simulink model "BMS_v1"  (R2024b)
settings: Solver=VariableStepAuto  StartTime=0.0  StopTime=1000  RelTol=1e-3  AbsTol=1e-3  EnableMultiTasking=on
libraries: fl_lib x30, nesl_utility x20, batt_lib x4
(part 2 of 2)

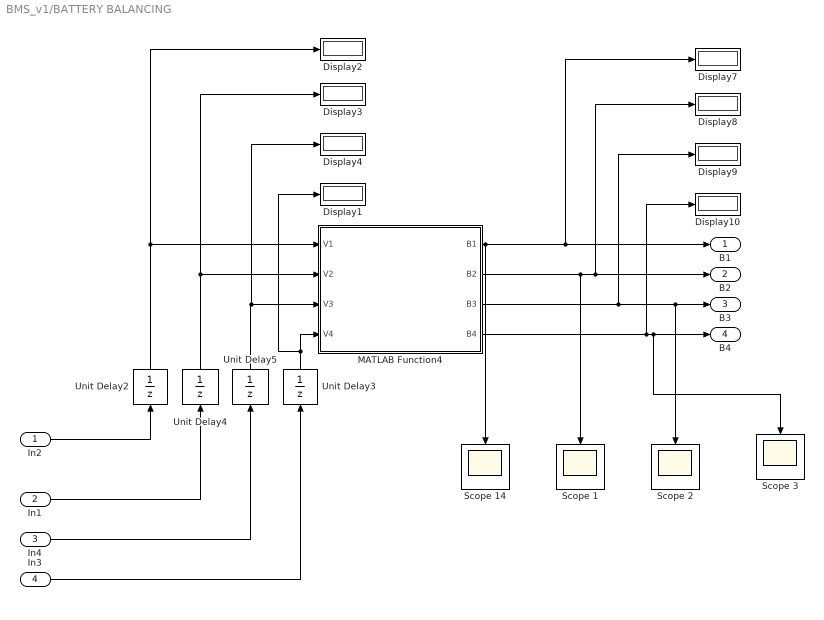
== system BMS_v1/BATTERY BALANCING ==
  In2 : Inport
  In1 : Inport  Port=2
  In4 : Inport  Port=3
  In3 : Inport  Port=4
  Display{1..4,7..10} (8 alike) : Display
  MATLAB Function4 : MATLAB Function  TreatAsAtomicUnit=on  SystemSampleTime=1
  Scope {1..3,14} (4 alike) : Scope
  Unit Delay{2..5} (4 alike) : UnitDelay  InitialCondition=4  HasFrameUpgradeWarning=on
  B1 : Outport
  B2 : Outport  Port=2
  B3 : Outport  Port=3
  B4 : Outport  Port=4
  wires:
  Unit Delay2/1 -> Display2/1, MATLAB Function4/1(V1)
  Unit Delay5/1 -> Display4/1, MATLAB Function4/3(V3)
  MATLAB Function4/4(B4) -> Scope 3/1, B4/1, Display10/1
  Unit Delay4/1 -> Display3/1, MATLAB Function4/2(V2)
  MATLAB Function4/2(B2) -> B2/1, Display8/1, Scope 1/1
  MATLAB Function4/1(B1) -> B1/1, Display7/1, Scope 14/1
  MATLAB Function4/3(B3) -> Scope 2/1, B3/1, Display9/1
  Unit Delay3/1 -> MATLAB Function4/4(V4), Display1/1
  In4/1 -> Unit Delay5/1
  In2/1 -> Unit Delay2/1
  In3/1 -> Unit Delay3/1
  In1/1 -> Unit Delay4/1

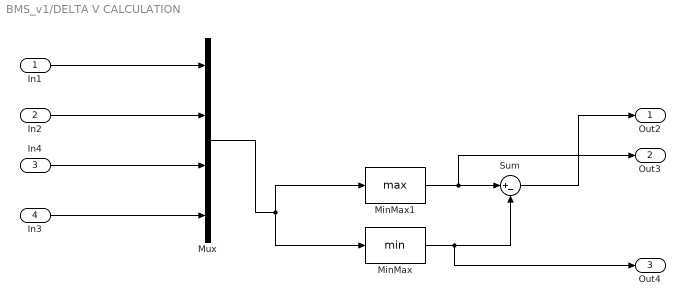
== system BMS_v1/DELTA V CALCULATION ==
  In1 : Inport
  In2 : Inport  Port=2
  In4 : Inport  Port=3
  In3 : Inport  Port=4
  MinMax : MinMax
  MinMax1 : MinMax  Function=max
  Mux : Mux
  Sum : Sum  Inputs=|+-
  Out2 : Outport
  Out3 : Outport  Port=2
  Out4 : Outport  Port=3
  wires:
  In3/1 -> Mux/4
  Mux/1 -> MinMax/1, MinMax1/1
  In1/1 -> Mux/1
  MinMax1/1 -> Out3/1, Sum/1
  MinMax/1 -> Out4/1, Sum/2
  In2/1 -> Mux/2
  Sum/1 -> Out2/1
  In4/1 -> Mux/3

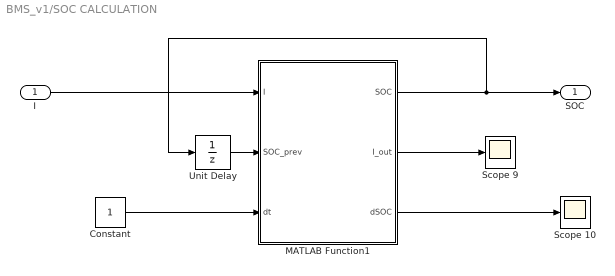
== system BMS_v1/SOC CALCULATION ==
  I : Inport
  Constant : Constant
  MATLAB Function1 : MATLAB Function  TreatAsAtomicUnit=on
  Scope 10 : Scope
  Scope 9 : Scope
  Unit Delay : UnitDelay  InitialCondition=0.9  HasFrameUpgradeWarning=on
  SOC : Outport
  wires:
  MATLAB Function1/1(SOC) -> SOC/1, Unit Delay/1
  MATLAB Function1/2(I_out) -> Scope 9/1
  MATLAB Function1/3(dSOC) -> Scope 10/1
  Constant/1 -> MATLAB Function1/3(dt)
  Unit Delay/1 -> MATLAB Function1/2(SOC_prev)
  I/1 -> MATLAB Function1/1(I)

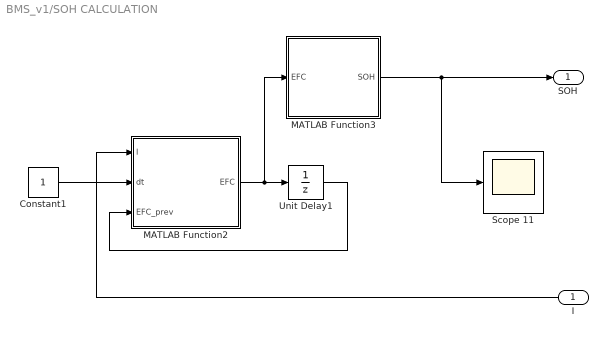
== system BMS_v1/SOH CALCULATION ==
  I : Inport
  Constant1 : Constant
  MATLAB Function2 : MATLAB Function  TreatAsAtomicUnit=on
  MATLAB Function3 : MATLAB Function  TreatAsAtomicUnit=on
  Scope 11 : Scope
  Unit Delay1 : UnitDelay  InitialCondition=0.9  HasFrameUpgradeWarning=on
  SOH : Outport
  wires:
  MATLAB Function2/1(EFC) -> MATLAB Function3/1(EFC), Unit Delay1/1
  MATLAB Function3/1(SOH) -> SOH/1, Scope 11/1
  Constant1/1 -> MATLAB Function2/2(dt)
  Unit Delay1/1 -> MATLAB Function2/3(EFC_prev)
  I/1 -> MATLAB Function2/1(I)

== matlab function BMS_v1/MATLAB Function3 ==
  data: Fault input; FaultCode input; State output; Reset input; System_Enable input; Charge_Request input; Discharge_Request input; Main_Contactor output; Precharge_Contactor output; Charge_Enable output; Discharge_Enable output; Fault_Action output; Precharge_Complete input; Time input
function [State, Main_Contactor, Precharge_Contactor, ...
          Charge_Enable, Discharge_Enable, Fault_Action] = ...
    BMS_State_Machine(Fault, FaultCode, Reset, System_Enable, ...
                      Charge_Request, Discharge_Request, ...
                      Precharge_Complete, Time)

% ============================================================
% BMS STATE MACHINE
%
% 0 = OFF
% 1 = INITIALIZE
% 2 = PRECHARGE
% 3 = IDLE
% 4 = CHARGING
% 5 = DISCHARGING
% 6 = FAULT
%
% Fault_Action:
% 0 = NORMAL
% 1 = WARNING / IMBALANCE
% 2 = CHARGE DISABLED
% 3 = DISCHARGE DISABLED
% 4 = CRITICAL FAULT
%
% FaultCode bits:
%
% 1   = Over-Voltage
% 2   = Under-Voltage
% 4   = Over-Current
% 8   = Over-Temperature
% 16  = Under-Temperature
% 32  = Cell Imbalance
% 64  = Low SOC
% 128 = Severe Fault
% 256 = Main Contactor Fault
% 512 = Precharge Contactor Fault
% ============================================================

persistent state
persistent precharge_start_time
persistent precharge_timeout_fault

if isempty(state)
    state = 0;
end

if isempty(precharge_start_time)
    precharge_start_time = 0;
end

if isempty(precharge_timeout_fault)
    precharge_timeout_fault = 0;
end

% ------------------------------------------------------------
% DEFAULT OUTPUTS
% ------------------------------------------------------------

State = 0;
Main_Contactor = 0;
Precharge_Contactor = 0;
Charge_Enable = 0;
Discharge_Enable = 0;
Fault_Action = 0;

% ------------------------------------------------------------
% FAULT CODE DECODING
% ------------------------------------------------------------

% Fault Manager uses uint16 because FaultCode can exceed 255
FC = uint16(FaultCode);

% Protection faults
OV   = bitand(FC,uint16(1))   ~= 0;
UV   = bitand(FC,uint16(2))   ~= 0;
OC   = bitand(FC,uint16(4))   ~= 0;
OT   = bitand(FC,uint16(8))   ~= 0;
UT   = bitand(FC,uint16(16))  ~= 0;
IMB  = bitand(FC,uint16(32))  ~= 0;
LSOC = bitand(FC,uint16(64))  ~= 0;
SEV  = bitand(FC,uint16(128)) ~= 0;

% Contactor diagnostic faults
MAIN_CONT_F  = bitand(FC,uint16(256)) ~= 0;
PRECH_CONT_F = bitand(FC,uint16(512)) ~= 0;

% ------------------------------------------------------------
% FAULT CLASSIFICATION
% ------------------------------------------------------------

if precharge_timeout_fault == 1

    % Latched precharge timeout
    Fault_Action = 4;

elseif Fault == 0

    Fault_Action = 0;

elseif SEV || OC || MAIN_CONT_F || PRECH_CONT_F

    % Critical faults
    Fault_Action = 4;

elseif OV || OT || UT

    % Charging prohibited
    Fault_Action = 2;

elseif UV || LSOC

    % Discharging prohibited
    Fault_Action = 3;

elseif IMB

    % Warning / balancing condition
    Fault_Action = 1;

else

    % Unknown fault = fail safe
    Fault_Action = 4;

end

% ============================================================
% STATE MACHINE
% ============================================================

switch state

    % ========================================================
    % STATE 0 : OFF
    % ========================================================

    case 0

        Main_Contactor = 0;
        Precharge_Contactor = 0;
        Charge_Enable = 0;
        Discharge_Enable = 0;

        precharge_start_time = 0;

        % Clear old timeout fault when system is completely OFF
        precharge_timeout_fault = 0;

        if System_Enable == 1

            state = 1;

        end


    % ========================================================
    % STATE 1 : INITIALIZE
    % ========================================================

    case 1

        Main_Contactor = 0;
        Precharge_Contactor = 0;
        Charge_Enable = 0;
        Discharge_Enable = 0;

        if Fault ~= 0

            state = 6;

        elseif precharge_timeout_fault == 1

            state = 6;

        else

            % Start precharge
            state = 2;

            % Record exact simulation time
            precharge_start_time = Time;

        end


    % ========================================================
    % STATE 2 : PRECHARGE
    % ========================================================

    case 2

        Precharge_Contactor = 1;
        Main_Contactor = 0;

        Charge_Enable = 0;
        Discharge_Enable = 0;

        % ----------------------------------------------------
        % CRITICAL FAULT DURING PRECHARGE
        % ----------------------------------------------------

        if Fault_Action == 4

            Precharge_Contactor = 0;
            Main_Contactor = 0;

            state = 6;

        % ----------------------------------------------------
        % PRECHARGE TIMEOUT
        % ----------------------------------------------------

        elseif (Time - precharge_start_time) >= 3

            Precharge_Contactor = 0;
            Main_Contactor = 0;

            % Latch timeout fault
            precharge_timeout_fault = 1;

            Fault_Action = 4;

            state = 6;

        % ----------------------------------------------------
        % PRECHARGE SUCCESS
        % ----------------------------------------------------

        elseif Precharge_Complete == 1

            Precharge_Contactor = 0;

            state = 3;

        end


    % ========================================================
    % STATE 3 : IDLE
    % ========================================================

    case 3

        Main_Contactor = 1;
        Precharge_Contactor = 0;

        Charge_Enable = 0;
        Discharge_Enable = 0;

        if Fault_Action == 4

            Main_Contactor = 0;

            state = 6;

        elseif Charge_Request == 1

            if Fault_Action ~= 2

                state = 4;

            end

        elseif Discharge_Request == 1

            if Fault_Action ~= 3

                state = 5;

            end

        end


    % ========================================================
    % STATE 4 : CHARGING
    % ========================================================

    case 4

        Main_Contactor = 1;
        Precharge_Contactor = 0;

        Charge_Enable = 1;
        Discharge_Enable = 0;

        if Fault_Action == 4

            Main_Contactor = 0;
            Charge_Enable = 0;

            state = 6;

        elseif Fault_Action == 2

            Charge_Enable = 0;

            state = 3;

        elseif Charge_Request == 0

            Charge_Enable = 0;

            state = 3;

        end


    % ========================================================
    % STATE 5 : DISCHARGING
    % ========================================================

    case 5

        Main_Contactor = 1;
        Precharge_Contactor = 0;

        Charge_Enable = 0;
        Discharge_Enable = 1;

        if Fault_Action == 4

            Main_Contactor = 0;
            Discharge_Enable = 0;

            state = 6;

        elseif Fault_Action == 3

            Discharge_Enable = 0;

            state = 3;

        elseif Discharge_Request == 0

            Discharge_Enable = 0;

            state = 3;

        end


    % ========================================================
    % STATE 6 : FAULT
    % ========================================================

    case 6

        Main_Contactor = 0;
        Precharge_Contactor = 0;
        Charge_Enable = 0;
        Discharge_Enable = 0;

        % ----------------------------------------------------
        % RECOVERY
        % ----------------------------------------------------

        if Reset == 1 && Fault == 0

            % Clear latched timeout fault
            precharge_timeout_fault = 0;

            state = 1;

        end


    % ========================================================
    % SAFETY DEFAULT
    % ========================================================

    otherwise

        state = 6;

        Main_Contactor = 0;
        Precharge_Contactor = 0;
        Charge_Enable = 0;
        Discharge_Enable = 0;

        Fault_Action = 4;

end

State = state;

end

== matlab function BMS_v1/MATLAB Function4 ==
  data: Protection_Fault input; Fault output; Protection_FaultCode input; Contactor_Fault input; Contactor_FaultCode input; FaultCode output
function [Fault, FaultCode] = ...
    BMS_FAULT_MANAGER(Protection_Fault, Protection_FaultCode, ...
                      Contactor_Fault, Contactor_FaultCode)

% ============================================================
% BMS FAULT MANAGER
%
% Combines protection faults and contactor diagnostic faults.
%
% Protection fault bits:
% 1   = Over-Voltage
% 2   = Under-Voltage
% 4   = Over-Current
% 8   = Over-Temperature
% 16  = Under-Temperature
% 32  = Cell Imbalance
% 64  = Low SOC
% 128 = Severe Protection Fault
%
% Contactor diagnostic bits:
% 256 = Main Contactor Fault
% 512 = Precharge Contactor Fault
% ============================================================

% ------------------------------------------------------------
% CONTACTOR FAULT DECODING
% ------------------------------------------------------------

Main_Contactor_Fault = ...
    bitand(uint8(Contactor_FaultCode),uint8(1)) ~= 0;

Precharge_Contactor_Fault = ...
    bitand(uint8(Contactor_FaultCode),uint8(2)) ~= 0;


% ------------------------------------------------------------
% SYSTEM FAULT
% ------------------------------------------------------------

Fault = Protection_Fault || ...
        Contactor_Fault;


% ------------------------------------------------------------
% SYSTEM FAULT CODE
% ------------------------------------------------------------

FaultCode = uint16(0);

% Preserve all existing protection bits
FaultCode = bitor(FaultCode, ...
                   uint16(Protection_FaultCode));


% Main contactor fault
if Main_Contactor_Fault

    FaultCode = bitor(FaultCode,uint16(256));

end


% Precharge contactor fault
if Precharge_Contactor_Fault

    FaultCode = bitor(FaultCode,uint16(512));

end

end

== matlab function BMS_v1/SOC CALCULATION/MATLAB Function1 ==
  data: I input; SOC output; SOC_prev input; dt input; I_out output; dSOC output
function [SOC, I_out, dSOC] = SOC_Estimator(I, SOC_prev, dt)

Qn = 2.5 * 3600;

dSOC = (I * dt) / Qn;

SOC = SOC_prev - dSOC;

SOC = min(max(SOC,0),1);

I_out = I;

== matlab function BMS_v1/SOH CALCULATION/MATLAB Function2 ==
  data: I input; EFC output; dt input; EFC_prev input
function EFC = EFC_Calculator(I, dt, EFC_prev)

Qn = 2.5 * 3600;     % Rated capacity in Coulombs

% Accumulated charge throughput
EFC = EFC_prev + abs(I) * dt / (2 * Qn);

end

== matlab function BMS_v1/SOH CALCULATION/MATLAB Function3 ==
  data: EFC input; SOH output
function SOH = SOH_Estimator(EFC)

Q_rated = 2.5;

% Demonstration degradation coefficient
k = 0.001;

Q_available = Q_rated * (1 - k * EFC);

SOH = Q_available / Q_rated;

SOH = min(max(SOH,0),1);

== matlab function BMS_v1/BATTERY BALANCING/MATLAB Function4 ==
  data: V1 input; B1 output; V2 input; V3 input; V4 input; B2 output; B3 output; B4 output
function [B1,B2,B3,B4] = Cell_Balancing(V1,V2,V3,V4)

% ============================================================
% STABLE PASSIVE CELL BALANCING
% 4S Li-ion battery
% ============================================================

persistent balance_cell
persistent timer
persistent balancing

if isempty(balance_cell)
    balance_cell = 0;
    timer = 0;
    balancing = false;
end

% ---- Parameters ----
V_ON  = 0.020;     % 20 mV: start balancing
V_OFF = 0.005;     % 5 mV: stop balancing

MIN_ON_TIME  = 300; % seconds
MIN_OFF_TIME = 60;  % seconds

% ---- Cell voltage vector ----
V = [V1 V2 V3 V4];

Vmax = max(V);
Vmin = min(V);
deltaV = Vmax - Vmin;

% ---- Default outputs ----
B1 = 0;
B2 = 0;
B3 = 0;
B4 = 0;

% ============================================================
% BALANCING CURRENTLY ACTIVE
% ============================================================

if balancing

    timer = timer + 1;

    % Keep the SAME cell ON until minimum ON time is reached
    if timer < MIN_ON_TIME

        if balance_cell == 1
            B1 = 1;
        elseif balance_cell == 2
            B2 = 1;
        elseif balance_cell == 3
            B3 = 1;
        elseif balance_cell == 4
            B4 = 1;
        end

        return;
    end

    % After minimum ON time, check whether balancing is finished
    Vcell = V(balance_cell);

    % Stop if this cell is sufficiently close to minimum
    if (Vcell - Vmin) <= V_OFF

        balancing = false;
        balance_cell = 0;
        timer = 0;

        return;
    end

    % If still high, continue balancing
    if balance_cell == 1
        B1 = 1;
    elseif balance_cell == 2
        B2 = 1;
    elseif balance_cell == 3
        B3 = 1;
    elseif balance_cell == 4
        B4 = 1;
    end

    return;
end

% ============================================================
% NO BALANCING CURRENTLY ACTIVE
% ============================================================

timer = timer + 1;

% Prevent immediate restart after switching OFF
if timer < MIN_OFF_TIME
    return;
end

% ============================================================
% START BALANCING ONLY IF IMBALANCE IS LARGE ENOUGH
% ============================================================

if deltaV >= V_ON

    % Find highest-voltage cell
    [~, balance_cell] = max(V);

    % Start balancing
    balancing = true;
    timer = 0;

    % Turn ON only the selected cell
    if balance_cell == 1
        B1 = 1;
    elseif balance_cell == 2
        B2 = 1;
    elseif balance_cell == 3
        B3 = 1;
    elseif balance_cell == 4
        B4 = 1;
    end
end

end

== matlab function BMS_v1/MATLAB Function1 ==
  data: V1 input; Fault output; V2 input; V3 input; V4 input; I input; T1 input; T2 input; T3 input; T4 input; SOC input; Reset input; FaultCode output; OV_Fault output; UV_Fault output; OC_Fault output; OT_Fault output; UT_Fault output; Imbalance_Fault output; LowSOC_Fault output
function [Fault,FaultCode,OV_Fault,UV_Fault,OC_Fault,...
         OT_Fault,UT_Fault,Imbalance_Fault,LowSOC_Fault] = ...
         BMS_PROTECTION(V1,V2,V3,V4,I,T1,T2,T3,T4,SOC,Reset)

% ============================================================
% BMS PROTECTION AND FAULT MANAGEMENT
% 4S Li-ion Battery
% ============================================================

% -------- Protection thresholds --------

CELL_OV = 4.20;          % Cell over-voltage
CELL_UV = 3.00;          % Cell under-voltage

CHARGE_OC    = 5.0;      % Charge over-current
DISCHARGE_OC = 10.0;     % Discharge over-current

TEMP_HIGH = 60;          % Over-temperature (deg C)
TEMP_LOW  = 0;           % Under-temperature (deg C)

IMBALANCE_LIMIT = 0.100; % 100 mV

SOC_LOW = 0.10;            % Low SOC (%)

% -------- Cell voltage vector --------

V = [V1 V2 V3 V4];

% -------- Temperature vector --------

T = [T1 T2 T3 T4];

% ============================================================
% INDIVIDUAL PROTECTION CONDITIONS
% ============================================================

% Over-voltage
OV_Fault = any(V >= CELL_OV);

% Under-voltage
UV_Fault = any(V <= CELL_UV);

% Current protection
if I > CHARGE_OC
    OC_Fault = 1;
elseif I < -DISCHARGE_OC
    OC_Fault = 1;
else
    OC_Fault = 0;
end

% Over-temperature
OT_Fault = any(T >= TEMP_HIGH);

% Under-temperature
UT_Fault = any(T <= TEMP_LOW);

% Cell imbalance
Vmax = max(V);
Vmin = min(V);

deltaV = Vmax - Vmin;

Imbalance_Fault = deltaV >= IMBALANCE_LIMIT;

% Low SOC
LowSOC_Fault = SOC <= SOC_LOW;

% ============================================================
% OVERALL FAULT
% ============================================================

Fault = OV_Fault || ...
        UV_Fault || ...
        OC_Fault || ...
        OT_Fault || ...
        UT_Fault || ...
        Imbalance_Fault || ...
        LowSOC_Fault;

% ============================================================
% 8-BIT FAULT CODE
% ============================================================

FaultCode = uint8(0);

% Bit 0 = Over-voltage
if OV_Fault
    FaultCode = bitor(FaultCode,uint8(1));
end

% Bit 1 = Under-voltage
if UV_Fault
    FaultCode = bitor(FaultCode,uint8(2));
end

% Bit 2 = Over-current
if OC_Fault
    FaultCode = bitor(FaultCode,uint8(4));
end

% Bit 3 = Over-temperature
if OT_Fault
    FaultCode = bitor(FaultCode,uint8(8));
end

% Bit 4 = Under-temperature
if UT_Fault
    FaultCode = bitor(FaultCode,uint8(16));
end

% Bit 5 = Cell imbalance
if Imbalance_Fault
    FaultCode = bitor(FaultCode,uint8(32));
end

% Bit 6 = Low SOC
if LowSOC_Fault
    FaultCode = bitor(FaultCode,uint8(64));
end

% Bit 7 = Reserved / severe fault
if Reset == 0 && (OV_Fault || UV_Fault || OT_Fault)
    FaultCode = bitor(FaultCode,uint8(128));
end

end

== matlab function BMS_v1/MATLAB Function2 ==
  data: Main_Command input; Main_Contactor_Fault output; Main_Feedback input; Precharge_Command input; Precharge_Feedback input; Time input; Precharge_Contactor_Fault output; Contactor_Fault output; Contactor_FaultCode output
function [Main_Contactor_Fault, Precharge_Contactor_Fault, ...
          Contactor_Fault, Contactor_FaultCode] = ...
    CONTACTOR_DIAGNOSTICS(Main_Command, Main_Feedback, ...
                          Precharge_Command, Precharge_Feedback, Time)

persistent main_mismatch_start
persistent precharge_mismatch_start
persistent main_fault
persistent precharge_fault

if isempty(main_mismatch_start)
    main_mismatch_start = -1;
end

if isempty(precharge_mismatch_start)
    precharge_mismatch_start = -1;
end

if isempty(main_fault)
    main_fault = 0;
end

if isempty(precharge_fault)
    precharge_fault = 0;
end

CONTACTOR_TIMEOUT = 0.1;

% ============================================================
% MAIN CONTACTOR
% ============================================================

main_mismatch = (Main_Command ~= Main_Feedback);

if main_mismatch

    if main_mismatch_start < 0
        main_mismatch_start = Time;
    end

    if (Time - main_mismatch_start) >= CONTACTOR_TIMEOUT
        main_fault = 1;
    end

else

    main_mismatch_start = -1;

end


% ============================================================
% PRECHARGE CONTACTOR
% ============================================================

precharge_mismatch = ...
    (Precharge_Command ~= Precharge_Feedback);

if precharge_mismatch

    if precharge_mismatch_start < 0
        precharge_mismatch_start = Time;
    end

    if (Time - precharge_mismatch_start) >= CONTACTOR_TIMEOUT
        precharge_fault = 1;
    end

else

    precharge_mismatch_start = -1;

end


% ============================================================
% OUTPUTS
% ============================================================

Main_Contactor_Fault = main_fault;
Precharge_Contactor_Fault = precharge_fault;

Contactor_Fault = main_fault || precharge_fault;

Contactor_FaultCode = uint8(0);

if main_fault
    Contactor_FaultCode = ...
        bitor(Contactor_FaultCode,uint8(1));
end

if precharge_fault
    Contactor_FaultCode = ...
        bitor(Contactor_FaultCode,uint8(2));
end

end
